simulink model "krstic_example_1p3"  (Simulink 10.1)
settings: Solver=ode45  StartTime=0.0  StopTime=100  RelTol=1e-3  EnableMultiTasking=on
settings Model: Creator=sbrunton  LastModifiedBy=Daniel
settings DataIOCC: LimitDataPoints=on  SignalLoggingSaveFormat=ModelDataLogs
settings OptimizationCC: ExpressionDepthLimit=2147483647
settings DebuggingCC: SolverPrmCheckMsg=warning  FcnCallInpInsideContextMsg=warning  StateNameClashWarn=warning

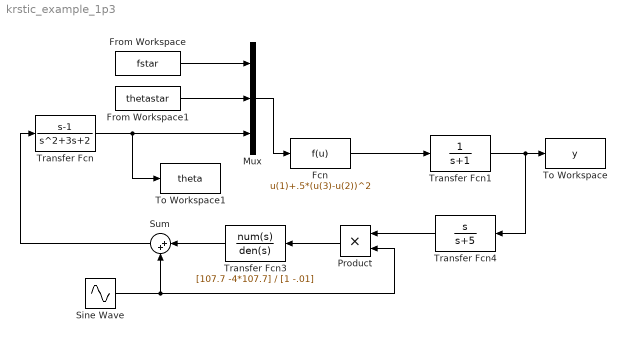
== system krstic_example_1p3 ==
  Fcn : Fcn  Expr=u(1)+.5*(u(3)-u(2))^2
  From Workspace : FromWorkspace  VariableName=fstar
  From Workspace1 : FromWorkspace  VariableName=thetastar
  Mux : Mux  Inputs=3
  Product : Product  RndMeth=Zero
  Sine Wave : Sin  Amplitude=.05  Frequency=5  SampleTime=0
  Sum : Sum  Inputs=|++
  To Workspace : ToWorkspace  VariableName=y  SampleTime=-1
  To Workspace1 : ToWorkspace  VariableName=theta  SampleTime=-1
  Transfer Fcn : TransferFcn  Numerator=[1 -1]  Denominator=[1 3 2]
  Transfer Fcn1 : TransferFcn  Denominator=[1 1]
  Transfer Fcn3 : TransferFcn  Numerator=[107.7 -4*107.7]  Denominator=[1 -.01]
  Transfer Fcn4 : TransferFcn  Numerator=[1 0]  Denominator=[1 5]
  wires:
  Transfer Fcn1/1 -> Transfer Fcn4/1, To Workspace/1
  Sum/1 -> Transfer Fcn/1
  From Workspace1/1 -> Mux/2
  From Workspace/1 -> Mux/1
  Transfer Fcn/1 -> Mux/3, To Workspace1/1
  Mux/1 -> Fcn/1
  Fcn/1 -> Transfer Fcn1/1
  Transfer Fcn4/1 -> Product/1
  Product/1 -> Transfer Fcn3/1
  Transfer Fcn3/1 -> Sum/1
  Sine Wave/1 -> Sum/2, Product/2
